simulink model "gleit_komma2"  (Simulink 7.8)
settings: Solver=ode45  StartTime=0.0  StopTime=100  RelTol=1e-3
settings Model: Creator=svenhoffmann  LastModifiedBy=josef  ExtModeAutoUpdateStatusClock=off
settings DataIOCC: SignalLoggingName=sigsOut
settings DebuggingCC: SaveWithParameterizedLinksMsg=none  SignalResolutionControl=TryResolveAllWithWarning  SolverPrmCheckMsg=none  MultiTaskDSMMsg=warning  MultiTaskCondExecSysMsg=none  StrictBusMsg=None
settings HardwareCC: TargetUnknown=on
settings RTWCC: IncludeERTFirstTime=on

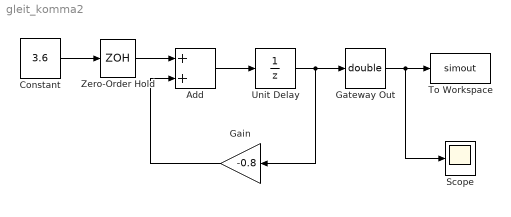
== system gleit_komma2 ==
  Add : Sum  OutDataTypeStr=single
  Constant : Constant  Value=3.6  OutDataTypeStr=single
  Gain : Gain  Gain=-0.8  OutDataTypeStr=Inherit: Same as input  ParamDataTypeStr=Inherit: Same as input
  Gateway Out : DataTypeConversion  OutDataTypeStr=double
  Scope : Scope
  To Workspace : ToWorkspace  VariableName=simout  SampleTime=-1  SaveFormat=Structure With Time
  Unit Delay : UnitDelay  X0=0.0  SampleTime=-1
  Zero-Order Hold : ZeroOrderHold
  wires:
  Constant/1 -> Zero-Order Hold/1
  Add/1 -> Unit Delay/1
  Unit Delay/1 -> Gateway Out/1, Gain/1
  Gain/1 -> Add/2
  Gateway Out/1 -> To Workspace/1, Scope/1
  Zero-Order Hold/1 -> Add/1
